simulink model "AC_long"  (R2026a)
settings: Solver=VariableStepAuto
values from neighbouring files (symbols this model uses):
  g = 9.81    [build_AC_long.m]
  M_alpha = A_V0(4,3)    [build_AC_long.m]
  M_dT = B_V0(4,2)    [build_AC_long.m]
  M_eta = B_V0(4,1)    [build_AC_long.m]
  M_q = A_V0(4,4)    [build_AC_long.m]
  M_V = A_V0(4,1) / V0    [build_AC_long.m]
  V0 = 200    [build_AC_long.m]
  x0 = [200; 0; 0; 0]    [check_AC_long.m]
  X_alpha = A_V0(1,3)    [build_AC_long.m]
  X_dT = B_V0(1,2) * V0    [build_AC_long.m]
  X_eta = B_V0(1,1) * V0    [build_AC_long.m]
  X_q = A_V0(1,4)    [build_AC_long.m]
  X_V = A_V0(1,1)    [build_AC_long.m]
  Z_alpha = mean([Z_alpha_a, Z_alpha_b])    [build_AC_long.m]
  Z_dT = mean([Z_dT_a, Z_dT_b])    [build_AC_long.m]
  Z_eta = mean([Z_eta_a, Z_eta_b])    [build_AC_long.m]
  Z_q = mean([Z_q_a, Z_q_b])    [build_AC_long.m]
  Z_V = mean([Z_V_a, Z_V_b])    [build_AC_long.m]
settings Model: Creator=devinbellll  LastModifiedBy=devinbellll

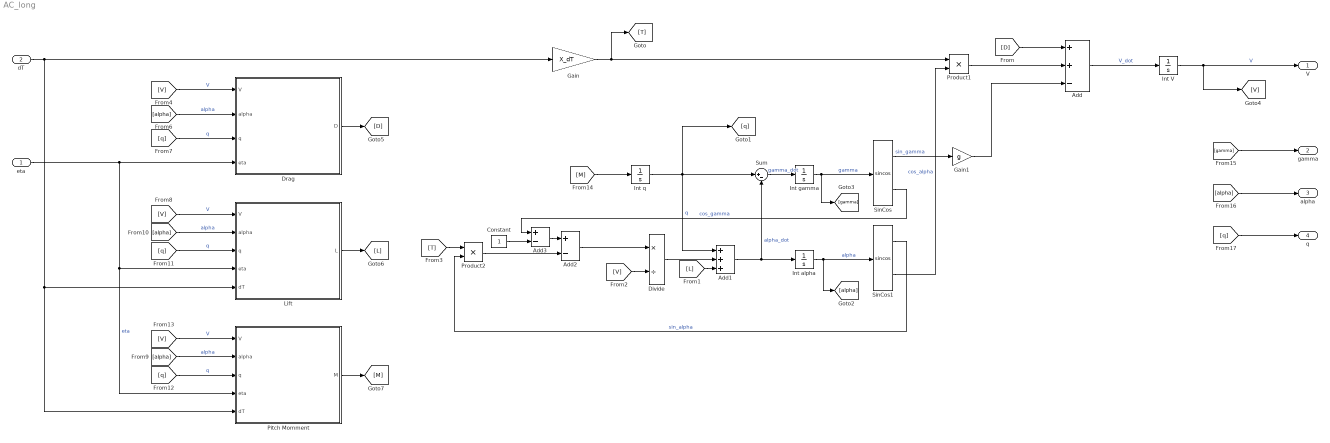
== system AC_long ==
  eta : Inport
  dT : Inport  Port=2
  Add : Sum  Inputs=++-
  Add1 : Sum  Inputs=+++
  Add2 : Sum  Inputs=+-
  Add3 : Sum  Inputs=+-
  Constant : Constant
  Divide : Product  Inputs=*/
  Drag : Subsystem
  Gain : Gain  Gain=X_dT
  Gain1 : Gain  Gain=g
  Int V : Integrator  InitialCondition=200
  Int alpha : Integrator  InitialCondition=x0(3)
  Int gamma : Integrator
  Int q : Integrator
  Lift : Subsystem
  Pitch Momment : Subsystem
  Product1 : Product
  Product2 : Product
  SinCos : Trigonometry  Operator=sincos
  SinCos1 : Trigonometry  Operator=sincos
  Sum : Sum  Inputs=|+-
  V : Outport
  gamma : Outport  Port=2
  alpha : Outport  Port=3
  q : Outport  Port=4
  wires:
  Int gamma/1 -> [gamma], SinCos/1  "gamma"
  Int alpha/1 -> [alpha], SinCos1/1  "alpha"
  SinCos/1 -> Gain1/1  "sin_gamma"
  SinCos/2 -> Add3/1  "cos_gamma"
  SinCos1/1 -> Product2/2  "sin_alpha"
  SinCos1/2 -> Product1/2  "cos_alpha"
  Sum/1 -> Int gamma/1  "gamma_dot"
  Add1/1 -> Int alpha/1, Sum/2  "alpha_dot"
  Int q/1 -> Add1/1, [q], Sum/1  "q"
  [M] -> Int q/1
  Int V/1 -> V/1, [V]  "V"
  Gain1/1 -> Add/3
  Gain/1 -> Product1/1, [T]
  Product1/1 -> Add/2
  Add/1 -> Int V/1  "V_dot"
  [D] -> Add/1
  [V] -> Divide/2
  Add2/1 -> Divide/1
  [L] -> Add1/3
  Divide/1 -> Add1/2
  [T] -> Product2/1
  [V] -> Drag/1(V)  "V"
  [alpha] -> Drag/2(alpha)  "alpha"
  [q] -> Drag/3(q)  "q"
  [q] -> Lift/3(q)  "q"
  [V] -> Lift/1(V)  "V"
  [alpha] -> Lift/2(alpha)  "alpha"
  Drag/1(D) -> [D]
  Lift/1(L) -> [L]
  [V] -> Pitch Momment/1(V)  "V"
  dT/1 -> Pitch Momment/5(dT), Lift/5(dT), Gain/1
  Pitch Momment/1(M) -> [M]
  [q] -> Pitch Momment/3(q)  "q"
  [alpha] -> Pitch Momment/2(alpha)  "alpha"
  eta/1 -> Drag/4(eta), Pitch Momment/4(eta), Lift/4(eta)  "eta"
  [gamma] -> gamma/1
  [alpha] -> alpha/1
  [q] -> q/1
  Product2/1 -> Add2/2
  Add3/1 -> Add2/1
  Constant/1 -> Add3/2

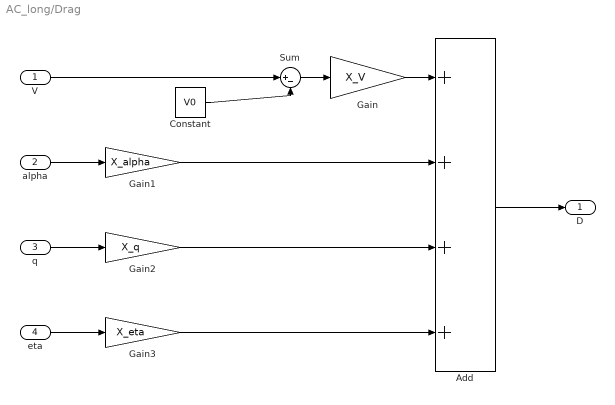
== system AC_long/Drag ==
  V : Inport
  alpha : Inport  Port=2
  q : Inport  Port=3
  eta : Inport  Port=4
  Add : Sum  Inputs=++++
  Constant : Constant  Value=V0
  Gain : Gain  Gain=X_V
  Gain1 : Gain  Gain=X_alpha
  Gain2 : Gain  Gain=X_q
  Gain3 : Gain  Gain=X_eta
  Sum : Sum  Inputs=|+-
  D : Outport
  wires:
  Constant/1 -> Sum/2
  Sum/1 -> Gain/1
  Gain/1 -> Add/1
  alpha/1 -> Gain1/1
  V/1 -> Sum/1
  Gain1/1 -> Add/2
  q/1 -> Gain2/1
  Gain2/1 -> Add/3
  eta/1 -> Gain3/1
  Gain3/1 -> Add/4
  Add/1 -> D/1

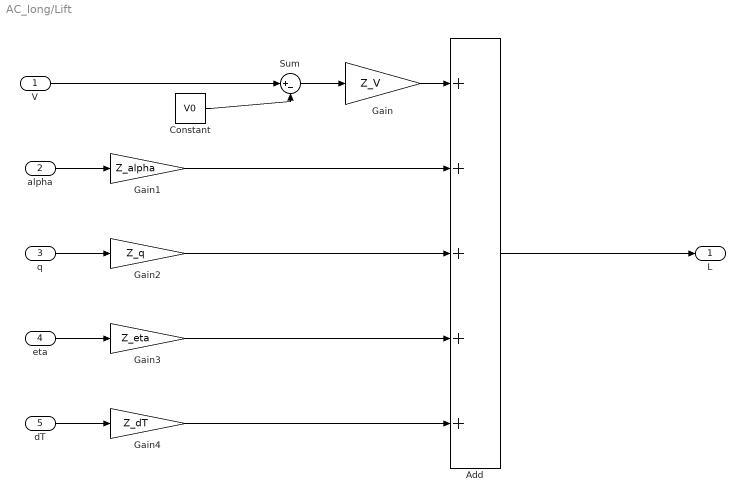
== system AC_long/Lift ==
  V : Inport
  alpha : Inport  Port=2
  q : Inport  Port=3
  eta : Inport  Port=4
  dT : Inport  Port=5
  Add : Sum  Inputs=+++++
  Constant : Constant  Value=V0
  Gain : Gain  Gain=Z_V
  Gain1 : Gain  Gain=Z_alpha
  Gain2 : Gain  Gain=Z_q
  Gain3 : Gain  Gain=Z_eta
  Gain4 : Gain  Gain=Z_dT
  Sum : Sum  Inputs=|+-
  L : Outport
  wires:
  V/1 -> Sum/1
  Gain3/1 -> Add/4
  alpha/1 -> Gain1/1
  Gain2/1 -> Add/3
  eta/1 -> Gain3/1
  Constant/1 -> Sum/2
  q/1 -> Gain2/1
  Sum/1 -> Gain/1
  Gain/1 -> Add/1
  dT/1 -> Gain4/1
  Gain4/1 -> Add/5
  Add/1 -> L/1
  Gain1/1 -> Add/2

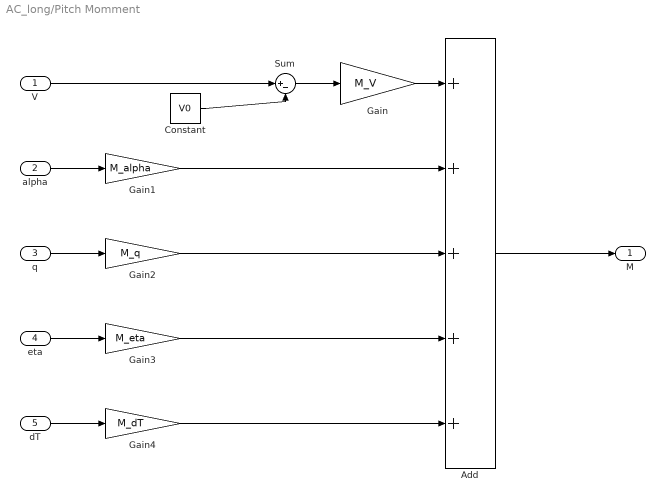
== system AC_long/Pitch Momment ==
  V : Inport
  alpha : Inport  Port=2
  q : Inport  Port=3
  eta : Inport  Port=4
  dT : Inport  Port=5
  Add : Sum  Inputs=+++++
  Constant : Constant  Value=V0
  Gain : Gain  Gain=M_V
  Gain1 : Gain  Gain=M_alpha
  Gain2 : Gain  Gain=M_q
  Gain3 : Gain  Gain=M_eta
  Gain4 : Gain  Gain=M_dT
  Sum : Sum  Inputs=|+-
  M : Outport
  wires:
  V/1 -> Sum/1
  Gain3/1 -> Add/4
  alpha/1 -> Gain1/1
  Gain2/1 -> Add/3
  eta/1 -> Gain3/1
  Gain1/1 -> Add/2
  Constant/1 -> Sum/2
  q/1 -> Gain2/1
  Sum/1 -> Gain/1
  Gain/1 -> Add/1
  dT/1 -> Gain4/1
  Gain4/1 -> Add/5
  Add/1 -> M/1
